simulink model "PB2M_001_007_RL"  (R2024a)
settings: Solver=FixedStepDiscrete  StartTime=0.0  StopTime=inf  FixedStep=[global_ST]  RelTol=1e-3
model workspace (MAT data in the model file):
  Var = 0
values from neighbouring files (symbols this model uses):
  global_ST = 1    [SimControl_v3_rl.m]    (also in SimControl_v4.m)
  global_time = [0:1:8784]'    [SimControl_v3_rl.m]    (also in SimControl_v4.m)
undefined symbols (not defined in the file or in its folder): acc, AEL, allActions, AMB, ATR, Bttry, CGH2, CGO2, CHP, COMPR, contActSpace, Ctrl, DiscIntNeverNeededParam, DIST, DRY, GASF, Gasf, imit_action_noise_variance, lowerLim, MES, NumEpisodes, NumImitLearning, numtraineps, PV, th, upperLim, vanilla, WT
libraries: simulink x1, rllib x1
(part 2 of 2)

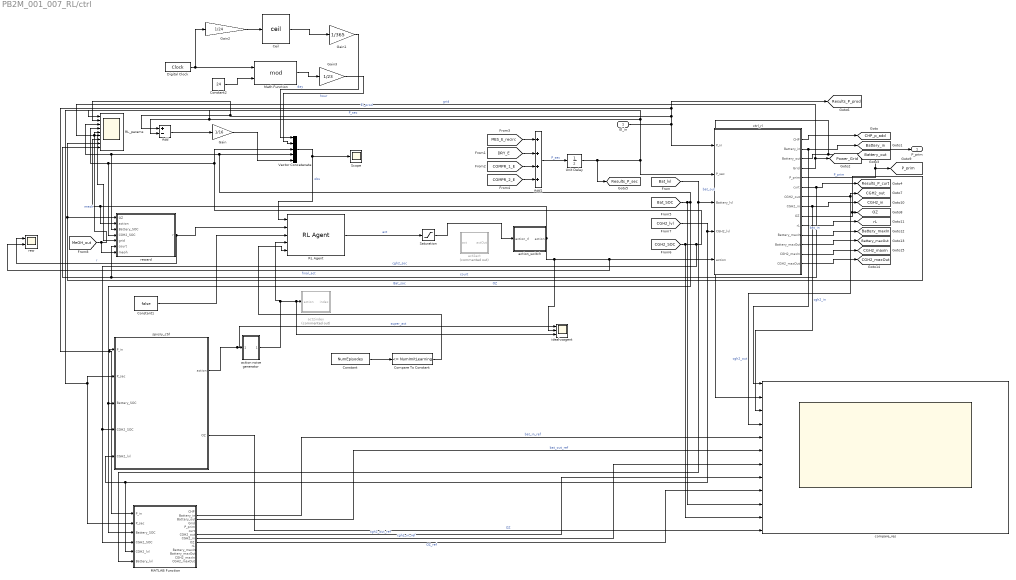
== system PB2M_001_007_RL/ctrl ==
  El_in : Inport
  Add : Sum  Inputs=+-
  Add1 : Sum  Inputs=++++
  Ceil : Rounding  Operator=ceil
  Compare To Constant : simulink/Logic and Bit Operations/Compare To Constant  relop=<=  const=NumImitLearning  OutDataTypeStr=boolean
  Constant : Constant  Value=NumEpisodes
  Constant1 : Constant  Value=false
  Constant2 : Constant  Value=24
  Digital Clock : DigitalClock
  Gain : Gain  Gain=1/16
  Gain1 : Gain  Gain=1/365
  Gain2 : Gain  Gain=1/24
  Gain3 : Gain  Gain=1/23
  MATLAB Function : MATLAB Function  TreatAsAtomicUnit=on
  Math Function : Math  Operator=mod
  RL Agent : rllib/RL Agent  Agent=agentObj  ExternalActionAsInput=on  ProvideLastAction=off  ProvideCumRwd=off  TreatAsDirectFeedthrough=on  UseStrictObservationDataTypes=off
  RL_params : Scope  NumInputPorts=9
  Saturation : Saturate  UpperLimit=upperLim  LowerLimit=lowerLim
  Scope : Scope
  Unit Delay : UnitDelay  SampleTime=-1  HasFrameUpgradeWarning=on
  Vector Concatenate : Concatenate  NumInputs=5
  act2act : MATLAB Function  Commented=on  TreatAsAtomicUnit=on
  act2index : MATLAB Function  Commented=on  TreatAsAtomicUnit=on
  action noise generator : Subsystem
  action_switch : Subsystem
  compare_res : Scope  NumInputPorts=12
  ctrl_rl : MATLAB Function  TreatAsAtomicUnit=on
  idealvsagent : Scope  NumInputPorts=3
  rew : Scope  NumInputPorts=2
  reward : MATLAB Function  TreatAsAtomicUnit=on
  spvsry_ctrl : MATLAB Function  TreatAsAtomicUnit=on
  P_prim : Outport
  tag scope: Battery_in=global, Battery_maxIn=global, Battery_maxOut=global, Battery_out=global, CGH2_in=global, CGH2_maxIn=global, CGH2_maxOut=global, CGH2_out=global, CHP_p_add=global, OZ=global, P_prim=global, Power_Grid=global, Results_P_curt=global, Results_P_prod=global, Results_P_sec=global, rL=global
  wires:
  [MES_E_recirc] -> Add1/1
  [DRY_E] -> Add1/2
  [COMPR_1_E] -> Add1/3
  [COMPR_2_E] -> Add1/4
  Add1/1 -> Unit Delay/1  "P_sec"
  ctrl_rl/5(P_prim) -> P_prim/1, [P_prim]  "P_prim"
  El_in/1 -> MATLAB Function/1(P_in), spvsry_ctrl/1(P_in), [Results_P_prod], RL_params/2, Add/1, ctrl_rl/1(P_in)  "El_prod"
  Unit Delay/1 -> [Results_P_sec], MATLAB Function/2(P_sec), spvsry_ctrl/2(P_sec), Add/2, RL_params/1, ctrl_rl/2(P_sec)  "P_sec"
  ctrl_rl/1(CHP) -> [CHP_p_add]
  ctrl_rl/2(Battery_in) -> compare_res/1, [Battery_in]  "bat_in"
  ctrl_rl/3(Battery_out) -> compare_res/2, [Battery_out]  "bat_out"
  ctrl_rl/4(Grid) -> reward/5(grid), RL_params/6, [Power_Grid]  "grid"
  ctrl_rl/6(curt) -> reward/6(court), RL_params/9, [Results_P_curt]  "court"
  ctrl_rl/7(CGH2_out) -> [CGH2_out], compare_res/4  "cgh2_out"
  ctrl_rl/9(OZ) -> RL_params/8, reward/1(OZ), [OZ]  "OZ"
  ctrl_rl/8(CGH2_in) -> compare_res/3, [CGH2_in]  "cgh2_in"
  ctrl_rl/10(rL) -> [rL]
  ctrl_rl/11(Battery_maxIn) -> [Battery_maxIn]
  ctrl_rl/12(Battery_maxOut) -> [Battery_maxOut]
  [Bat_lvl] -> MATLAB Function/6(Battery_lvl), ctrl_rl/3(Battery_lvl)
  [CGH2_SOC] -> compare_res/11, MATLAB Function/4(CGH2_SOC), spvsry_ctrl/4(CGH2_SOC), Vector Concatenate/3, RL_params/4, reward/4(CGH2_SOC)  "cgh2_soc"
  [Bat_SOC] -> compare_res/10, reward/3(Battery_SOC), RL_params/3, Vector Concatenate/4, MATLAB Function/3(Battery_SOC), spvsry_ctrl/3(Battery_SOC)  "Bat_soc"
  ctrl_rl/14(CGH2_maxOut) -> [CGH2_maxOut]
  ctrl_rl/13(CGH2_maxIn) -> [CGH2_maxIn]
  [CGH2_lvl] -> spvsry_ctrl/5(CGH2_lvl), MATLAB Function/5(CGH2_lvl), ctrl_rl/4(CGH2_lvl)
  Vector Concatenate/1 -> Scope/1, RL Agent/1  "obs"
  [MeOH_out] -> reward/7(meoh), RL_params/5  "meoh"
  reward/1(r) -> rew/1, RL Agent/2  "r"
  Compare To Constant/1 -> RL Agent/5
  Constant/1 -> Compare To Constant/1
  spvsry_ctrl/1(action) -> idealvsagent/1, action noise generator/1(action)  "super_act"
  Constant1/1 -> RL Agent/3
  action_switch/1(action) -> idealvsagent/2, rew/2, ctrl_rl/5(action), RL_params/7, reward/2(action)  "final_act"
  Digital Clock/1 -> Gain2/1, Math Function/1
  Gain2/1 -> Ceil/1
  Constant2/1 -> Math Function/2
  Ceil/1 -> Gain1/1
  Gain1/1 -> Vector Concatenate/1  "day"
  Math Function/1 -> Gain3/1
  Gain3/1 -> Vector Concatenate/2  "hour"
  RL Agent/1 -> Saturation/1  "act"
  action noise generator/1(Out1) -> RL Agent/4, idealvsagent/3, act2index/1(action)
  Saturation/1 -> action_switch/1(action_rl)
  Add/1 -> Gain/1
  Gain/1 -> Vector Concatenate/5
  MATLAB Function/2(Battery_in) -> compare_res/5  "bat_in_ref"
  MATLAB Function/3(Battery_out) -> compare_res/6  "bat_out_ref"
  MATLAB Function/8(CGH2_in) -> compare_res/7  "cgh2_in_ref"
  MATLAB Function/7(CGH2_out) -> compare_res/8  "cgh2_out_ref"
  MATLAB Function/9(OZ) -> compare_res/9  "OZ_ref"
  spvsry_ctrl/2(OZ) -> compare_res/12  "OZ"

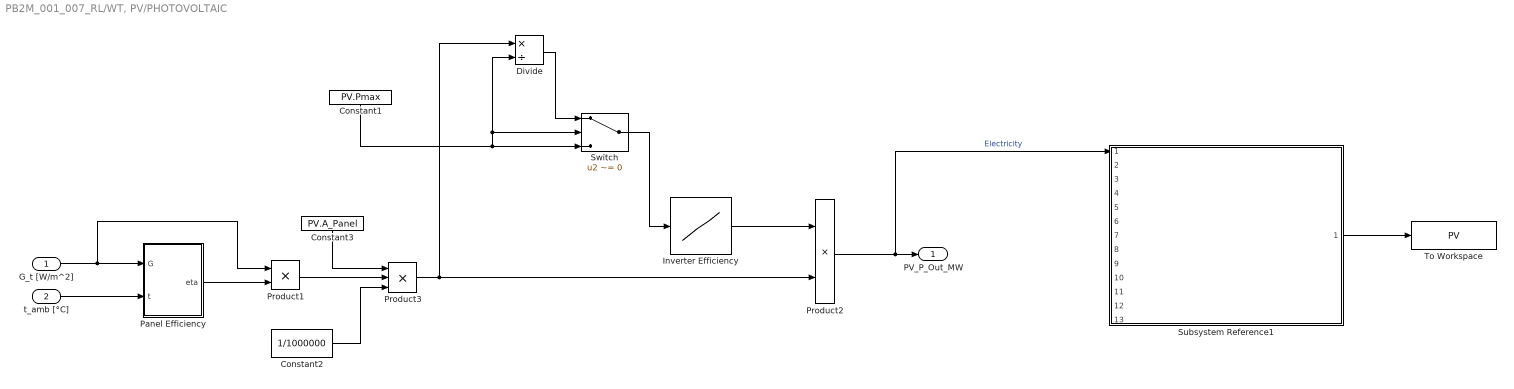
== system PB2M_001_007_RL/WT, PV/PHOTOVOLTAIC ==
  G_t [W/m^2] : Inport
  t_amb [°C] : Inport  Port=2
  Constant1 : Constant  Value=PV.Pmax
  Constant2 : Constant  Value=1/1000000
  Constant3 : Constant  Value=PV.A_Panel
  Divide : Product  Inputs=*/
  Inverter Efficiency : Lookup_n-D  NumberOfTableDimensions=1  BreakpointsForDimension1=[PV.Inv_LU.P_relat]'  Table=[PV.Inv_LU.eta_inv]'  InternalRulePriority=Speed  RndMeth=Simplest
  Panel Efficiency : MATLAB Function  TreatAsAtomicUnit=on
  Product1 : Product
  Product2 : Product
  Product3 : Product  Inputs=3
  Subsystem Reference1 : Subsystem  ReferencedSubsystem=PB2M_RltHub_002
  Switch : Switch  Criteria=u2 ~= 0  SaturateOnIntegerOverflow=off  InputSameDT=off
  To Workspace : ToWorkspace  VariableName=PV  SampleTime=-1
  PV_P_Out_MW : Outport
  wires:
  G_t [W/m^2]/1 -> Panel Efficiency/1(G), Product1/1
  t_amb [°C]/1 -> Panel Efficiency/2(t)
  Panel Efficiency/1(eta) -> Product1/2
  Product1/1 -> Product3/2
  Inverter Efficiency/1 -> Product2/1
  Product2/1 -> Subsystem Reference1/1, PV_P_Out_MW/1  "Electricity"
  Constant3/1 -> Product3/1
  Constant2/1 -> Product3/3
  Product3/1 -> Divide/1, Product2/2
  Divide/1 -> Switch/1
  Switch/1 -> Inverter Efficiency/1
  Constant1/1 -> Divide/2, Switch/2, Switch/3
  Subsystem Reference1/1 -> To Workspace/1

== system PB2M_001_007_RL/WT, PV/WIND TURBINE ==
  v_wind [m/s] : Inport
  Add : Sum
  Constant : Constant  Value=WT.n_typeA
  Constant1 : Constant  Value=WT.n_typeB
  Constant2 : Constant  Value=WT.ws_corr_factor
  Product : Product
  Product1 : Product
  Product2 : Product
  Subsystem Reference1 : Subsystem  ReferencedSubsystem=PB2M_RltHub_002
  To Workspace1 : ToWorkspace  VariableName=WT  SampleTime=-1
  V112 3.45 MW : Lookup_n-D  NumberOfTableDimensions=1  BreakpointsForDimension1=[WT.PowerCurve.v_wind]'  Table=[WT.PowerCurve.P_WT_3_45]'  InternalRulePriority=Speed  RndMeth=Simplest
  V112 4.2 MW : Lookup_n-D  NumberOfTableDimensions=1  BreakpointsForDimension1=[WT.PowerCurve.v_wind]'  Table=[WT.PowerCurve.P_WT_4_2]'  InternalRulePriority=Speed  RndMeth=Simplest
  WT_P_Out [MW] : Outport
  wires:
  V112 3.45 MW/1 -> Product/2
  Constant/1 -> Product/1
  V112 4.2 MW/1 -> Product1/1
  Constant1/1 -> Product1/2
  Product/1 -> Add/1
  Product1/1 -> Add/2
  Add/1 -> Subsystem Reference1/1, WT_P_Out [MW]/1  "Electricity"
  v_wind [m/s]/1 -> Product2/1
  Product2/1 -> V112 3.45 MW/1, V112 4.2 MW/1
  Constant2/1 -> Product2/2
  Subsystem Reference1/1 -> To Workspace1/1

== system PB2M_001_007_RL/ctrl/action noise generator ==
  action : Inport
  Add : Sum
  Random Number : RandomNumber  Variance=imit_action_noise_variance  Seed=[NumEpisodes NumEpisodes+numtraineps]  SampleTime=1
  Saturation : Saturate  UpperLimit=1  LowerLimit=-1
  Out1 : Outport
  wires:
  Add/1 -> Saturation/1
  Random Number/1 -> Add/2
  action/1 -> Add/1
  Saturation/1 -> Out1/1

== system PB2M_001_007_RL/ctrl/action_switch ==
  action_rl : Inport
  Constant8 : Constant  Value=vanilla  SampleTime=1
  Multiport Switch : MultiPortSwitch  DataPortOrder=Specify indices  DataPortIndices={0,1,2,3}  SaturateOnIntegerOverflow=off  InputSameDT=off
  Switch Case : SwitchCase  CaseConditions={0,1,2,3}  ShowDefaultCase=off
  Switch Case Action Subsystem : Subsystem  TreatAsAtomicUnit=on
  Switch Case Action Subsystem1 : Subsystem  TreatAsAtomicUnit=on
  Switch Case Action Subsystem2 : Subsystem  TreatAsAtomicUnit=on
  Switch Case Action Subsystem3 : Subsystem  TreatAsAtomicUnit=on
  action : Outport
  wires:
  Switch Case Action Subsystem1/1(Out1) -> Multiport Switch/3
  Constant8/1 -> Multiport Switch/1, Switch Case/1
  Switch Case/4 -> Switch Case Action Subsystem3/Action
  Switch Case Action Subsystem/1(action) -> Multiport Switch/2
  Switch Case/3 -> Switch Case Action Subsystem2/Action
  Switch Case/1 -> Switch Case Action Subsystem/Action
  Switch Case/2 -> Switch Case Action Subsystem1/Action
  Switch Case Action Subsystem2/1(Out1) -> Multiport Switch/4
  Switch Case Action Subsystem3/1(Out1) -> Multiport Switch/5
  action_rl/1 -> Switch Case Action Subsystem/1(In1)
  Multiport Switch/1 -> action/1

== system PB2M_001_007_RL/ctrl/action_switch/Switch Case Action Subsystem ==
  In1 : Inport
  Action Port : ActionPort  ActionPortLabel=case [ 0 ]:
  action : Outport
  wires:
  In1/1 -> action/1

== system PB2M_001_007_RL/ctrl/action_switch/Switch Case Action Subsystem1 ==
  Action Port : ActionPort  ActionPortLabel=case [ 1 ]:
  Constant : Constant  Value=[-1 -1]
  Out1 : Outport
  wires:
  Constant/1 -> Out1/1

== system PB2M_001_007_RL/ctrl/action_switch/Switch Case Action Subsystem2 ==
  Action Port : ActionPort  ActionPortLabel=case [ 2 ]:
  Uniform Random Number : UniformRandomNumber  Minimum=[-1 -1]  Maximum=[1 1]  Seed=[0 1]  SampleTime=1
  Out1 : Outport
  wires:
  Uniform Random Number/1 -> Out1/1

== system PB2M_001_007_RL/ctrl/action_switch/Switch Case Action Subsystem3 ==
  Action Port : ActionPort  ActionPortLabel=case [ 3 ]:
  Constant : Constant  Value=[0,0]
  Out1 : Outport
  wires:
  Constant/1 -> Out1/1

== matlab function PB2M_001_007_RL/ctrl/reward ==
  data: OZ input; r output; action input; Battery_SOC input; CGH2_SOC input; grid input; court input; meoh input
function r = rewardfcn(OZ, action, Battery_SOC, CGH2_SOC, grid, court, meoh)
if court || grid
    r = -grid/20 -court/20;
else
    r = meoh;
end


% sigma = 0.1;
% act_bat = action(2);
% act_cgh = action(1);
% mu1 = 0;
% mu2 = 0;
%     % r1 = 0.5 * sqrt(2*pi) * sigma * normpdf(act_bat,mu1,sigma);
%     % r2 = 0.5 * sqrt(2*pi) * sigma * normpdf(act_cgh,mu2,sigma);
%     % r = r1 + r2;
% if OZ == 2
%         switch true
%             case Battery_SOC > 0.9
%                 mu1 = 0.3;
%             case Battery_SOC > 0.8
%                 mu1 = 0.1;
%             case Battery_SOC < 0.3
%                 mu1 = -0.075;
%             case Battery_SOC < 0.4
%                mu1 = -0.05;
%             case Battery_SOC < 0.5
%                 mu1 = -0.025;
%         end
%         r1 = 0.5 * sqrt(2*pi) * sigma * normpdf(act_bat,mu1,sigma);
% 
%         switch true
%             case CGH2_SOC > 0.9
%                 mu2 = 0.3;
%             case CGH2_SOC > 0.8
%                 mu2 = 0.2;
%             case CGH2_SOC < 0.3
%                 mu2 = -0.075;
%             case CGH2_SOC < 0.4
%                 mu2 = -0.05;
%             case CGH2_SOC < 0.5
%                 mu2 = -0.025;
%         end
%         r2 = 0.5 * sqrt(2*pi) * sigma * normpdf(act_cgh,mu2,sigma);
% 
% 
% else 
%     r1 = 0.5 * sqrt(2*pi) * sigma * normpdf(act_bat,mu1,sigma);
%     r2 = 0.5 * sqrt(2*pi) * sigma * normpdf(act_cgh,mu2,sigma);
% end
%     r = r1 + r2;
% end

== matlab function PB2M_001_007_RL/BM /MATLAB Function ==
  data: mflow_H2 input; module output; mflow_SG input; th parameter; ATR parameter
function module = module_calc(mflow_H2, mflow_SG, th, ATR)
module = module_calc_ex(mflow_H2, mflow_SG, th, ATR);

end

== matlab function PB2M_001_007_RL/ctrl/spvsry_ctrl ==
  data: P_in input; action output; P_sec input; Battery_SOC input; CGH2_SOC input; Ctrl parameter; AEL parameter; Gasf parameter; OZ output; CGH2_lvl input; CGH2 parameter
function [action,OZ]  = supervisory_control(P_in, P_sec, Battery_SOC, CGH2_SOC, Ctrl, AEL, Gasf, CGH2_lvl, CGH2)

P_prim = P_in - P_sec; % P prim ist die theoretische Leistung, die für den Elektrolyseur zur Verfügung ist. Überschüsse und Mängel werden ausgeglichen, damit der Elektrolyseur innerhalb seiner Lastgrenzen fahren kann
rL = P_prim / AEL.Pmax; % rL ist der theoretische relative Load, in dem die Anlage fahren würde, wenn keine Hilfsssysteme (Grid, Speicher, CHP) genutzt werden
action = [0 0];
OZ = 0;

CGH2_maxIn     = (CGH2.Cap - CGH2_lvl) / 3.6; 
CGH2_maxOut    = (CGH2_lvl - CGH2.min) / 3.6;

% Battery_maxIn  = Bttry.Cap - Battery_lvl;
% Battery_maxOut = Battery_lvl - Bttry.min;


%% CASES
switch true
    case rL < AEL.rLmin
        OZ = 0;
        max_act1 = -CGH2_maxOut / ((Gasf.rLmax-AEL.rLmin)*AEL.Pmax*Ctrl.AEL.fac);
        action(1) = -(Gasf.rLmin-AEL.rLmin)/(Gasf.rLmax-AEL.rLmin);
        action(1) = max(max_act1,action(1));
        action(1) = min(action(1),0);
        action(2) = -((Gasf.rLmin-rL) + action(1)*(Gasf.rLmax-AEL.rLmin));

    case AEL.rLmin <= rL && rL < Gasf.rLmin
        OZ = 1;
        max_act1 = -CGH2_maxOut / ((Gasf.rLmax-AEL.rLmin)*AEL.Pmax*Ctrl.AEL.fac);
        action(1) = -(Gasf.rLmin-rL)/(Gasf.rLmax-AEL.rLmin);
        action(1) = max(max_act1,action(1));
        action(1) = min(action(1),0);
        action(2) = -((Gasf.rLmin-rL) + action(1)*(Gasf.rLmax-AEL.rLmin));

    case rL >= Gasf.rLmin && rL <= Gasf.rLmax
        OZ = 2;
        switch true
            case Battery_SOC > 0.9
                action(2) = -0.3*P_prim/AEL.Pmax;
            case Battery_SOC > 0.8
                action(2) = -0.1*P_prim/AEL.Pmax;
            case Battery_SOC < 0.3
                action(2) = 0.075*P_prim/AEL.Pmax;
            case Battery_SOC < 0.4
                action(2) = 0.05*P_prim/AEL.Pmax;
            case Battery_SOC < 0.5
                action(2) = 0.025*P_prim/AEL.Pmax;
        end

        switch true
            case CGH2_SOC > 0.9
                action(1) = -0.3*P_prim/((Gasf.rLmax-AEL.rLmin)*AEL.Pmax);
            case CGH2_SOC > 0.8
                action(1) = -0.1*P_prim/((Gasf.rLmax-AEL.rLmin)*AEL.Pmax);
            case CGH2_SOC < 0.3
                action(1) = 0.075*P_prim/((AEL.rLmax-Gasf.rLmin)*AEL.Pmax);
            case CGH2_SOC < 0.4
                action(1) = 0.05*P_prim/((AEL.rLmax-Gasf.rLmin)*AEL.Pmax);
            case CGH2_SOC < 0.5
                action(1) = 0.025*P_prim/((AEL.rLmax-Gasf.rLmin)*AEL.Pmax);
        end

    case Gasf.rLmax < rL && rL <= AEL.rLmax
        OZ = 3;
        action(1) = (rL-Gasf.rLmax) / (AEL.rLmax-Gasf.rLmin);
        max_act1 = CGH2_maxIn / ((AEL.rLmax-Gasf.rLmin)*AEL.Pmax*Ctrl.AEL.fac);
        action(1) = min(action(1),max_act1);
        action(1) = max(action(1),0);
        action(2) = (rL -Gasf.rLmax) - action(1)*(AEL.rLmax-Gasf.rLmin);

    case rL > AEL.rLmax
        OZ = 4;
        action(1) = (AEL.rLmax-Gasf.rLmax) / (AEL.rLmax-Gasf.rLmin);
        max_act1 = CGH2_maxIn / ((AEL.rLmax-Gasf.rLmin)*AEL.Pmax*Ctrl.AEL.fac);
        action(1) = min(action(1),max_act1);
        action(1) = max(action(1),0);
        action(2) = (rL -Gasf.rLmax) - action(1)*(AEL.rLmax-Gasf.rLmin);
end

== matlab function PB2M_001_007_RL/BM /Ideal Controller ==
  data: fac input; CHP input; Hydrogen input; GASF parameter; DRY parameter; ATR parameter; BM_wet output
function BM_wet = biopath(fac, CHP, Hydrogen, GASF, DRY, ATR)
BM_wet = biopath_ex(Hydrogen, fac, CHP, ATR, GASF, DRY);
end

== matlab function PB2M_001_007_RL/ctrl/act2act ==
  data: act input; actOut output; allActions parameter; contActSpace parameter
function actOut = act2mat(act,allActions,contActSpace)
if contActSpace
    actvec = linspace(0,1,size(allActions, 1));
    diff = abs(actvec-act);
    [~,action] = min(diff);
    actOut = allActions(action,:);
else
    actOut = allActions(act,:);
end

== matlab function PB2M_001_007_RL/ctrl/act2index ==
  data: action input; index output; allActions parameter; acc parameter; contActSpace parameter
function index = act2index(action, allActions, acc, contActSpace)
index = act2index(allActions, action, acc, contActSpace);

end

== matlab function PB2M_001_007_RL/ctrl/MATLAB Function ==
  data: P_in input; CHP output; P_sec input; Battery_SOC input; CGH2_SOC input; Battery_in output; Battery_out output; Grid output; P_prim output; curt output; CGH2_out output; CGH2_in output; OZ output; rL output; Battery_maxIn output; Battery_maxOut output; CGH2_maxIn output; CGH2_maxOut output; Bttry parameter; Gasf parameter; AEL parameter; Ctrl parameter; CGH2 parameter; CGH2_lvl input; Battery_lvl input
function [CHP, Battery_in, Battery_out, Grid, P_prim, curt, CGH2_out, CGH2_in, OZ, rL, Battery_maxIn, Battery_maxOut, CGH2_maxIn, CGH2_maxOut] = manage_power_ex_v8(P_in, P_sec, Battery_SOC, CGH2_SOC, Bttry, Gasf, AEL, Ctrl, CGH2, CGH2_lvl,Battery_lvl)

persistent bit_bttry

%% Initialsierung

if isempty(bit_bttry)
    bit_bttry = 1;
end

Battery_in = 0;
Battery_out = 0;
CHP = 0;
Grid = 0;
curt = 0;
CGH2_in = 0;
CGH2_out = 0;
OZ = 0;


P_prim = P_in - P_sec; % P prim ist die theoretische Leistung, die für den Elektrolyseur zur Verfügung ist. Überschüsse und Mängel werden ausgeglichen, damit der Elektrolyseur innerhalb seiner Lastgrenzen fahren kann
rL = P_prim / AEL.Pmax; % rL ist der theoretische relative Load, in dem die Anlage fahren würde, wenn keine Hilfsssysteme (Grid, Speicher, CHP) genutzt werden


CGH2_maxIn     = (CGH2.Cap - CGH2_lvl) / 3.6;
CGH2_maxOut    = (CGH2_lvl - CGH2.min) / 3.6;

Battery_maxIn  = Bttry.Cap - Battery_lvl;
Battery_maxOut = Battery_lvl - Bttry.min;



%% Überprüfung ob Batterie leer ist

if Battery_lvl <= (Bttry.min + 0.01 * Bttry.Cap)
    bit_bttry = 0;
elseif Battery_lvl >= Bttry.Cap / 2
    bit_bttry = 1;
end


%% CASES
switch true
    case rL < AEL.rLmin
        OZ = 0;
        CGH2_out = min((Gasf.rLmin - AEL.rLmin) * AEL.Pmax * Ctrl.AEL.fac, CGH2_maxOut);
        CGH2_out = max(CGH2_out,0);
        Battery_out= min((Gasf.rLmin - rL) * AEL.Pmax - CGH2_out / Ctrl.AEL.fac, Battery_maxOut);
        Battery_out = max(Battery_out,0);
        Grid = (Gasf.rLmin - rL) * AEL.Pmax - CGH2_out / Ctrl.AEL.fac - Battery_out;      

    case AEL.rLmin <= rL && rL < Gasf.rLmin
        OZ = 1;
        CGH2_out = min((Gasf.rLmin - rL) * AEL.Pmax * Ctrl.AEL.fac, CGH2_maxOut);
        CGH2_out = max(CGH2_out,0);
        Battery_out = min((Gasf.rLmin - rL) * AEL.Pmax - CGH2_out / Ctrl.AEL.fac, Battery_maxOut);
        Battery_out = max(Battery_out,0);
        Grid = (Gasf.rLmin - rL) * AEL.Pmax - CGH2_out / Ctrl.AEL.fac - Battery_out;

    case rL >= Gasf.rLmin && rL <= Gasf.rLmax
        OZ = 2;
        switch true
            case Battery_SOC > 0.9
                Battery_out = min([0.3 * P_prim, Battery_maxOut]);
            case Battery_SOC > 0.8
                Battery_out = min([0.1 * P_prim,Battery_maxOut]);
            case Battery_SOC < 0.3
                Battery_in = min([0.075 * P_prim, Battery_maxIn]);
            case Battery_SOC < 0.4
                Battery_in = min([0.05 * P_prim,Battery_maxIn]);
            case Battery_SOC < 0.5
                Battery_in = min([0.025 * P_prim,Battery_maxIn]);
        end

        switch true
            case CGH2_SOC > 0.9
                CGH2_out = min([0.3 * P_prim * Ctrl.AEL.fac, CGH2_maxOut]);
            case CGH2_SOC > 0.8
                CGH2_out = min([0.1 * P_prim * Ctrl.AEL.fac, CGH2_maxOut]);
            case CGH2_SOC < 0.3
                CGH2_in = min([0.075 * P_prim * Ctrl.AEL.fac,  CGH2_maxIn]);
            case CGH2_SOC < 0.4
                CGH2_in = min([0.05 * P_prim * Ctrl.AEL.fac, CGH2_maxIn]);
            case CGH2_SOC < 0.5
                CGH2_in = min([0.025 * P_prim * Ctrl.AEL.fac, CGH2_maxIn]);
        end
            
    case Gasf.rLmax < rL && rL <= AEL.rLmax
        OZ = 3;
        CGH2_in = min((rL - Gasf.rLmax) * AEL.Pmax * Ctrl.AEL.fac, CGH2_maxIn);
        CGH2_in = max(CGH2_in,0);
        Battery_in = min(((rL - Gasf.rLmax) * AEL.Pmax - CGH2_in / Ctrl.AEL.fac), Battery_maxIn);
        Battery_in = max(Battery_in, 0);% Ist der H2 Speicher voll, müssen wir den AEL runterregeln, indem wir die Batterie laden
        curt = P_prim - AEL.Pmax - CGH2_in / Ctrl.AEL.fac - Battery_in;

    case rL > AEL.rLmax
        OZ = 4;
        CGH2_in =    min((AEL.rLmax - Gasf.rLmax) * AEL.Pmax * Ctrl.AEL.fac, CGH2_maxIn);
        CGH2_in = max(CGH2_in,0);
        Battery_in = min((rL - Gasf.rLmax) * AEL.Pmax - CGH2_in / Ctrl.AEL.fac, Battery_maxIn);
        Battery_in = max(Battery_in, 0);
        curt = P_prim - AEL.Pmax - CGH2_in / Ctrl.AEL.fac - Battery_in;

end

end

== stateflow chart PB2M_001_007_RL/O2 Distribution/O2_DISTRIBUTION ==
  state ACTION
    O2_req = SMR_req + GASF_req;
    shortage = O2_req - AEL_act;
    CGO2_maxIn = (CGO2_cap - CGO2_lvl) * 1000 / 720;
    CGO2_maxOut = CGO2_lvl * 1000 / 720;
    state Surplus
      CGO2_out = 0;
      CGO2_in = min(abs(shortage), CGO2_maxIn);
      SMR = SMR_req;
      GASF = GASF_req;
    state Shortage
      CGO2_out = min(shortage, CGO2_maxOut);
      CGO2_in = 0;
      SMR = SMR_req;
      GASF = GASF_req;
    (default) -> Shortage
    Shortage -> Surplus : [shortage <= 0]
    Surplus -> Shortage : [shortage > 0]
  data: SMR_req input; AEL_act input; CGO2_in output; CGO2_out output; SMR output; O2_req local; shortage local; CGO2_lvl input; CGO2_cap constant double =CGO2.Cap; CGO2_maxIn local; CGO2_maxOut local; GASF_req input; GASF output

== matlab function PB2M_001_007_RL/WT, PV/PHOTOVOLTAIC/Panel Efficiency ==
  data: G input; eta output; t input; PV parameter
function eta = TotalEff(G, t, PV)

eta = PV_PanelEff_Ex(G, t, PV);

end

== matlab function PB2M_001_007_RL/ctrl/ctrl_rl ==
  data: CHP output; Battery_in output; P_in input; P_sec input; Battery_lvl input; CGH2_lvl input; Battery_out output; Grid output; P_prim output; curt output; Bttry parameter; CGH2 parameter; AEL parameter; Gasf parameter; CGH2_out output; CGH2_in output; OZ output; Ctrl parameter; rL output; Battery_maxIn output; Battery_maxOut output; CGH2_maxIn output; CGH2_maxOut output; action input
% function [CHP, Battery_in, Battery_out, Grid, P_prim, curt, CGH2_out, CGH2_in, OZ, rL, Battery_maxIn, Battery_maxOut, CGH2_maxIn, CGH2_maxOut] = manage_power_ex_v8_RL(P_in, P_sec, Battery_lvl, CGH2_lvl, Bttry, CGH2, AEL, Gasf, Ctrl, action)
% 
% persistent bit_bttry
% 
% %% Initialsierung
% 
% if isempty(bit_bttry)
%     bit_bttry = 1;
% end
% 
% Battery_in = 0;
% Battery_out = 0;
% CHP = 0;
% Grid = 0;
% curt = 0;
% CGH2_in = 0;
% CGH2_out = 0;
% OZ = 0;
% act_cgh2 = action(1);
% act_bat = action(2);
% 
% 
% P_prim = P_in - P_sec; % P prim ist die theoretische Leistung, die für den Elektrolyseur zur Verfügung ist. Überschüsse und Mängel werden ausgeglichen, damit der Elektrolyseur innerhalb seiner Lastgrenzen fahren kann
% rL = P_prim / AEL.Pmax; % rL ist der theoretische relative Load, in dem die Anlage fahren würde, wenn keine Hilfsssysteme (Grid, Speicher, CHP) genutzt werden
% 
% 
% CGH2_maxIn     = (CGH2.Cap - CGH2_lvl) / 3.6;
% CGH2_maxOut    = (CGH2_lvl - CGH2.min) / 3.6;
% 
% Battery_maxIn  = Bttry.Cap - Battery_lvl;
% Battery_maxOut = Battery_lvl - Bttry.min;
% 
% 
% 
% %% Überprüfung ob Batterie leer ist
% 
% if Battery_lvl <= (Bttry.min + 0.01 * Bttry.Cap)
%     bit_bttry = 0;
% elseif Battery_lvl >= Bttry.Cap / 2
%     bit_bttry = 1;
% end
% 
% 
% %% CASES
% switch true
%     case rL < AEL.rLmin
%         OZ = 0;
%         CGH2_out = min((Gasf.rLmin - AEL.rLmin) * AEL.Pmax * Ctrl.AEL.fac, CGH2_maxOut);
%         Bat0_1 = min((Gasf.rLmin - AEL.rLmin) * AEL.Pmax - CGH2_out / Ctrl.AEL.fac, Battery_maxOut);
%         Bat0_2 = min((AEL.rLmin - rL) * AEL.Pmax, Battery_maxOut - Bat0_1);
%         Battery_out = Bat0_1 + Bat0_2;
%         Grid = (Gasf.rLmin - rL) * AEL.Pmax - CGH2_out / Ctrl.AEL.fac - Battery_out;      
% 
%     case AEL.rLmin <= rL && rL < Gasf.rLmin
%         OZ = 1;
%         CGH2_out = min((Gasf.rLmin - rL) * AEL.Pmax * Ctrl.AEL.fac, CGH2_maxOut);
%         Battery_out = min((Gasf.rLmin - rL) * AEL.Pmax - CGH2_out / Ctrl.AEL.fac, Battery_maxOut);
%         Grid = (Gasf.rLmin - rL) * AEL.Pmax - CGH2_out / Ctrl.AEL.fac - Battery_out;
% 
%     case rL >= Gasf.rLmin && rL <= Gasf.rLmax
%         OZ = 2;
%         switch true
%             case act_bat >= 0
%                 Battery_out = min([act_bat * P_prim, 0.45 * (Gasf.rLmax - rL) * AEL.Pmax, Battery_maxOut]);
%             case act_bat < 0
%                 Battery_in = min([-act_bat * P_prim, 0.45 * (rL - Gasf.rLmin) * AEL.Pmax, Battery_maxIn]);  % act_bat (-1,1)
%         end
% 
%         switch true
%             case act_cgh2 >= 0
%                 CGH2_out = min([act_cgh2 * P_prim, 0.45 * (Gasf.rLmax - rL) * AEL.Pmax * Ctrl.AEL.fac, CGH2_maxOut]);
%             case act_cgh2 < 0
%                 CGH2_in = min([-act_cgh2 * P_prim, 0.45 * (rL - Gasf.rLmin) * AEL.Pmax * Ctrl.AEL.fac, CGH2_maxIn]); % act_cgh2(-1,1)
%         end
% 
%     case Gasf.rLmax < rL && rL <= AEL.rLmax
%         OZ = 3;
%         CGH2_in = min((rL - Gasf.rLmax) * AEL.Pmax * Ctrl.AEL.fac, CGH2_maxIn);
%         Battery_in = min(((rL - Gasf.rLmax) * AEL.Pmax - CGH2_in / Ctrl.AEL.fac), Battery_maxIn); % Ist der H2 Speicher voll, müssen wir den AEL runterregeln, indem wir die Batterie laden
%         curt = P_prim - AEL.Pmax - CGH2_in / Ctrl.AEL.fac - Battery_in;
% 
%     case rL > AEL.rLmax
%         OZ = 4;
%         CGH2_in =    min((AEL.rLmax - Gasf.rLmax) * AEL.Pmax * Ctrl.AEL.fac, CGH2_maxIn);
%         Bat4_1 = min((AEL.rLmax - Gasf.rLmax) * AEL.Pmax - CGH2_in / Ctrl.AEL.fac, Battery_maxIn);
%         Bat4_2 = min((rL - AEL.rLmax) * AEL.Pmax, Battery_maxIn - Bat4_1);
%         Battery_in = Bat4_1 + Bat4_2;
%         curt = P_prim - AEL.Pmax - CGH2_in / Ctrl.AEL.fac - Battery_in;
% end
% end

% function [CHP, Battery_in, Battery_out, Grid, P_prim, curt, CGH2_out, CGH2_in, OZ, rL, Battery_maxIn, Battery_maxOut, CGH2_maxIn, CGH2_maxOut] = manage_power_ex_v8(P_in, P_sec, Battery_lvl, Battery_SOC, CGH2_lvl, CGH2_SOC, Bttry, CGH2, AEL, Gasf, Ctrl, chp, action)
% 
% persistent bit_bttry
% 
% %% Initialsierung
% 
% if isempty(bit_bttry)
%     bit_bttry = 1;
% end
% 
% Battery_in = 0;
% Battery_out = 0;
% CHP = 0;
% Grid = 0;
% curt = 0;
% CGH2_in = 0;
% CGH2_out = 0;
% OZ = 0;
% 
% 
% P_prim = P_in - P_sec; % P prim ist die theoretische Leistung, die für den Elektrolyseur zur Verfügung ist. Überschüsse und Mängel werden ausgeglichen, damit der Elektrolyseur innerhalb seiner Lastgrenzen fahren kann
% rL = P_prim / AEL.Pmax; % rL ist der theoretische relative Load, in dem die Anlage fahren würde, wenn keine Hilfsssysteme (Grid, Speicher, CHP) genutzt werden
% 
% 
% CGH2_maxIn     = (CGH2.Cap - CGH2_lvl) / 3.6;
% CGH2_maxOut    = (CGH2_lvl - CGH2.min) / 3.6;
% 
% Battery_maxIn  = Bttry.Cap - Battery_lvl;
% Battery_maxOut = Battery_lvl - Bttry.min;
% 
% 
% 
% %% Überprüfung ob Batterie leer ist
% 
% if Battery_lvl <= (Bttry.min + 0.01 * Bttry.Cap)
%     bit_bttry = 0;
% elseif Battery_lvl >= Bttry.Cap / 2
%     bit_bttry = 1;
% end
% 
% 
% %% CASES
% switch true
%     case rL < AEL.rLmin
%         OZ = 0;
%         CGH2_out = min((Gasf.rLmin - AEL.rLmin) * AEL.Pmax * Ctrl.AEL.fac, CGH2_maxOut);
%         Bat0_1 = min((Gasf.rLmin - AEL.rLmin) * AEL.Pmax - CGH2_out / Ctrl.AEL.fac, Battery_maxOut);
%         Bat0_2 = min((AEL.rLmin - rL) * AEL.Pmax, Battery_maxOut - Bat0_1);
%         Battery_out = Bat0_1 + Bat0_2;
%         Grid = (Gasf.rLmin - rL) * AEL.Pmax - CGH2_out / Ctrl.AEL.fac - Battery_out;      
% 
%     case AEL.rLmin <= rL && rL < Gasf.rLmin
%         OZ = 1;
%         CGH2_out = min((Gasf.rLmin - rL) * AEL.Pmax * Ctrl.AEL.fac, CGH2_maxOut);
%         Battery_out = min((Gasf.rLmin - rL) * AEL.Pmax - CGH2_out / Ctrl.AEL.fac, Battery_maxOut);
%         Grid = (Gasf.rLmin - rL) * AEL.Pmax - CGH2_out / Ctrl.AEL.fac - Battery_out;
% 
%     case rL >= Gasf.rLmin && rL <= Gasf.rLmax
%         OZ = 2;
%         switch true
%             case Battery_SOC > 0.9
%                 Battery_out = min([0.3 * P_prim, 0.45 * (Gasf.rLmax - rL) * AEL.Pmax, Battery_maxOut]);
%             case Battery_SOC > 0.8
%                 Battery_out = min([0.1 * P_prim, 0.45 * (Gasf.rLmax - rL) * AEL.Pmax, Battery_maxOut]);
%             case Battery_SOC < 0.3
%                 Battery_in = min([0.075 * P_prim, 0.45 * (rL - Gasf.rLmin) * AEL.Pmax, Battery_maxIn]);
%             case Battery_SOC < 0.4
%                 Battery_in = min([0.05 * P_prim, 0.45 * (rL - Gasf.rLmin) * AEL.Pmax, Battery_maxIn]);
%             case Battery_SOC < 0.5
%                 Battery_in = min([0.025 * P_prim, 0.45 * (rL - Gasf.rLmin) * AEL.Pmax, Battery_maxIn]);
%         end
% 
%         switch true
%             case CGH2_SOC > 0.9
%                 CGH2_out = min([0.3 * P_prim, 0.45 * (Gasf.rLmax - rL) * AEL.Pmax * Ctrl.AEL.fac, CGH2_maxOut]);
%             case CGH2_SOC > 0.8
%                 CGH2_out = min([0.1 * P_prim, 0.45 * (Gasf.rLmax - rL) * AEL.Pmax * Ctrl.AEL.fac, CGH2_maxOut]);
%             case CGH2_SOC < 0.3
%                 CGH2_in = min([0.075 * P_prim, 0.45 * (rL - Gasf.rLmin) * AEL.Pmax * Ctrl.AEL.fac, CGH2_maxIn]);
%             case CGH2_SOC < 0.4
%                 CGH2_in = min([0.05 * P_prim, 0.45 * (rL - Gasf.rLmin) * AEL.Pmax * Ctrl.AEL.fac, CGH2_maxIn]);
%             case CGH2_SOC < 0.5
%                 CGH2_in = min([0.025 * P_prim, 0.45 * (rL - Gasf.rLmin) * AEL.Pmax * Ctrl.AEL.fac, CGH2_maxIn]);
%         end
% 
%     case Gasf.rLmax < rL && rL <= AEL.rLmax
%         OZ = 3;
%         CGH2_in = min((rL - Gasf.rLmax) * AEL.Pmax * Ctrl.AEL.fac, CGH2_maxIn);
%         Battery_in = min(((rL - Gasf.rLmax) * AEL.Pmax - CGH2_in / Ctrl.AEL.fac), Battery_maxIn); % Ist der H2 Speicher voll, müssen wir den AEL runterregeln, indem wir die Batterie laden
%         curt = P_prim - AEL.Pmax - CGH2_in / Ctrl.AEL.fac - Battery_in;
% 
%     case rL > AEL.rLmax
%         OZ = 4;
%         CGH2_in =    min((AEL.rLmax - Gasf.rLmax) * AEL.Pmax * Ctrl.AEL.fac, CGH2_maxIn);
%         Bat4_1 = min((AEL.rLmax - Gasf.rLmax) * AEL.Pmax - CGH2_in / Ctrl.AEL.fac, Battery_maxIn);
%         Bat4_2 = min((rL - AEL.rLmax) * AEL.Pmax, Battery_maxIn - Bat4_1);
%         Battery_in = Bat4_1 + Bat4_2;
%         curt = P_prim - AEL.Pmax - CGH2_in / Ctrl.AEL.fac - Battery_in;
% end
% end

function [CHP, Battery_in, Battery_out, Grid, P_prim, curt, CGH2_out, CGH2_in, OZ, rL, Battery_maxIn, Battery_maxOut, CGH2_maxIn, CGH2_maxOut] = manage_power_ex_v8_RL(P_in, P_sec, Battery_lvl, CGH2_lvl, Bttry, CGH2, AEL, Gasf, Ctrl, action)


Battery_in = 0;
Battery_out = 0;
CHP = 0;
Grid = 0;
curt = 0;
CGH2_in = 0;
CGH2_out = 0;
OZ = 0;
act_cgh = action(1);
act_bat = action(2);


P_prim = P_in - P_sec; % P prim ist die theoretische Leistung, die für den Elektrolyseur zur Verfügung ist. Überschüsse und Mängel werden ausgeglichen, damit der Elektrolyseur innerhalb seiner Lastgrenzen fahren kann
rL = P_prim / AEL.Pmax; % rL ist der theoretische relative Load, in dem die Anlage fahren würde, wenn keine Hilfsssysteme (Grid, Speicher, CHP) genutzt werden


CGH2_maxIn     = (CGH2.Cap - CGH2_lvl) / 3.6; 
CGH2_maxOut    = (CGH2_lvl - CGH2.min) / 3.6;

Battery_maxIn  = Bttry.Cap - Battery_lvl;
Battery_maxOut = Battery_lvl - Bttry.min;


switch true
    case act_cgh < 0
        CGH2_out = min(-act_cgh * (Gasf.rLmax - AEL.rLmin) * AEL.Pmax * Ctrl.AEL.fac, CGH2_maxOut);
        CGH2_out = max(CGH2_out,0);
    case act_cgh >= 0
        CGH2_in = min(act_cgh * (AEL.rLmax - Gasf.rLmin) * AEL.Pmax * Ctrl.AEL.fac, CGH2_maxIn);
        CGH2_in = max(CGH2_in,0);
end

switch true 
    case act_bat < 0
        Battery_out = min(-act_bat * AEL.Pmax, Battery_maxOut);
        Battery_out = max(Battery_out,0);

    case act_bat >= 0
        Battery_in = min(act_bat * AEL.Pmax, Battery_maxIn);
        Battery_in = max(Battery_in, 0);
end

curt = max(P_prim + CGH2_out + Battery_out - AEL.Pmax - CGH2_in / Ctrl.AEL.fac - Battery_in,0);
Grid = max((Gasf.rLmin - rL) * AEL.Pmax + CGH2_in/Ctrl.AEL.fac + Battery_in - CGH2_out / Ctrl.AEL.fac - Battery_out,0); 

end
